simulink model "VSI_o_loop_Gid"  (Simulink 8.2)
settings: Solver=ode23t  StartTime=0.0  StopTime=0.5  MaxStep=25e-6  RelTol=1e-4  AbsTol=1e-5
values from neighbouring files (symbols this model uses):
  C = 1*31.5e-6    (= 3.15e-05)    [TVSI_vil_tf_cal_sim_comp_frd_model.m]    (also in VSI_ol_init.m = 3.13e-05; VSI_ol_tf_cal_sim_comp_frd_model.m = 3.13e-05; Zac_VSI.m = 3.18e-05; Zdc_VSI.m)
  Dd = 0.29997    [TVSI_vil_tf_cal_sim_comp_frd_model.m]    (also in VSI_ol_init.m = 0.299645524555; VSI_ol_tf_cal_sim_comp_frd_model.m = 0.367252524302; Zac_VSI.m = 0.3674)
  Dq = 0.08    [TVSI_vil_tf_cal_sim_comp_frd_model.m]    (also in VSI_ol_init.m = 0.0661607498065; VSI_ol_tf_cal_sim_comp_frd_model.m = 0.000664512470614; Zac_VSI.m = 0.0012)
  L = 1.0e-3    (= 0.001)    [TVSI_vil_tf_cal_sim_comp_frd_model.m]    (also in VSI_ol_init.m; VSI_ol_tf_cal_sim_comp_frd_model.m; Zac_VSI.m = 0.000506643235509; Zdc_VSI.m)
  R = 12    [TVSI_vil_tf_cal_sim_comp_frd_model.m]    (also in VSI_ol_init.m = 15; VSI_ol_tf_cal_sim_comp_frd_model.m = 12000; Zac_VSI.m; Zdc_VSI.m)
  RL = 0.13    [TVSI_vil_tf_cal_sim_comp_frd_model.m]    (also in VSI_ol_init.m = 0.15; VSI_ol_tf_cal_sim_comp_frd_model.m = 0.15; Zac_VSI.m = 0.06; Zdc_VSI.m)
  Vdc = 270    [TVSI_vil_tf_cal_sim_comp_frd_model.m]    (also in VSI_ol_init.m; VSI_ol_tf_cal_sim_comp_frd_model.m; Zac_VSI.m; Zdc_VSI.m)
  w = 500*2*pi    (= 3141.59265359)    [JF_CMOD.m]    (also in JF_SMOD.m; TVSI_vil_tf_cal_sim_comp_frd_model.m = 376.991118431; VSI_ol_init.m = 2513.27412287; VSI_ol_tf_cal_sim_comp_frd_model.m = 376.991118431)
libraries: powerlib x22
settings Model: Creator=marko  LastModifiedBy=wenbo  BufferReuse=off
settings OptimizationCC: BlockReduction=off  InlineParams=on  BufferReuse=off
settings DebuggingCC: AlgebraicLoopMsg=none  SolverPrmCheckMsg=none  UnconnectedInputMsg=none  UnconnectedOutputMsg=none  UnconnectedLineMsg=none

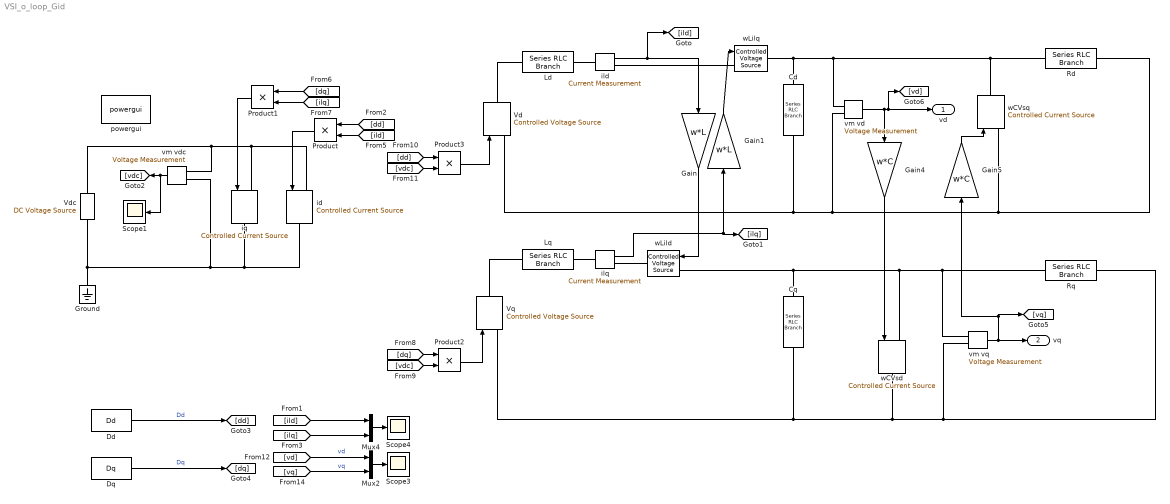
== system VSI_o_loop_Gid ==
  Cd : powerlib/Elements/Series RLC Branch  LConnTagsString=__new0  RConnTagsString=__new0  BranchType=C  Resistance=1  Inductance=1e-3  SetiL0=off  InitialCurrent=0  Capacitance=C  Setx0=off  InitialVoltage=0  Measurements=None
  Cq : powerlib/Elements/Series RLC Branch  LConnTagsString=__new0  RConnTagsString=__new0  BranchType=C  Resistance=1  Inductance=1e-3  SetiL0=off  InitialCurrent=0  Capacitance=C  Setx0=off  InitialVoltage=0  Measurements=None
  Dd : Constant  Value=Dd
  Dq : Constant  Value=Dq
  Gain : Gain  Gain=w*L
  Gain1 : Gain  Gain=w*L
  Gain4 : Gain  Gain=w*C
  Gain5 : Gain  Gain=w*C
  Ground : powerlib/Elements/Ground  LConnTagsString=a
  Ld : powerlib/Elements/Series RLC Branch  LConnTagsString=__new0  RConnTagsString=__new0  BranchType=RL  Resistance=RL  Inductance=L  SetiL0=off  InitialCurrent=0  Capacitance=1e-6  Setx0=off  InitialVoltage=0  Measurements=None
  Lq : powerlib/Elements/Series RLC Branch  LConnTagsString=__new0  RConnTagsString=__new0  BranchType=RL  Resistance=RL  Inductance=L  SetiL0=off  InitialCurrent=0  Capacitance=1e-6  Setx0=off  InitialVoltage=0  Measurements=None
  Mux2 : Mux  Inputs=2
  Mux4 : Mux  Inputs=2
  Product{,1..3} (4 alike) : Product  RndMeth=Zero
  Rd : powerlib/Elements/Series RLC Branch  LConnTagsString=__new0  RConnTagsString=__new0  BranchType=R  Resistance=R  Inductance=1e-3  SetiL0=off  InitialCurrent=0  Capacitance=1e-6  Setx0=off  InitialVoltage=0  Measurements=None
  Rq : powerlib/Elements/Series RLC Branch  LConnTagsString=__new0  RConnTagsString=__new0  BranchType=R  Resistance=R  Inductance=1e-3  SetiL0=off  InitialCurrent=0  Capacitance=1e-6  Setx0=off  InitialVoltage=0  Measurements=None
  Scope1 : Scope
      settings: YMin=270  YMax=270  SaveName=ildq_matlab
  Scope3 : Scope
      settings: YMin=-0.25  YMax=5.25  SaveName=ildq_matlab2
  Scope4 : Scope
      settings: YMin=-0.25  YMax=5.25  SaveName=ildq_matlab1
  Vd : powerlib/Electrical Sources/Controlled Voltage Source  Initialize=on  Source_Type=DC  Amplitude=0  Phase=0  Frequency=0  Measurements=None
  Vdc : powerlib/Electrical Sources/DC Voltage Source  Amplitude=Vdc  Measurements=None
  Vq : powerlib/Electrical Sources/Controlled Voltage Source  Initialize=on  Source_Type=DC  Amplitude=0  Phase=0  Frequency=0  Measurements=None
  id : powerlib/Electrical Sources/Controlled Current Source  Initialize=on  Source_Type=DC  Amplitude=0  Phase=0  Frequency=0  Measurements=None
  ild : powerlib/Measurements/Current Measurement  PhasorSimulation=off  OutputType=Complex  PSBequivalent=0
  ilq : powerlib/Measurements/Current Measurement  PhasorSimulation=off  OutputType=Complex  PSBequivalent=0
  iq : powerlib/Electrical Sources/Controlled Current Source  Initialize=on  Source_Type=DC  Amplitude=0  Phase=0  Frequency=0  Measurements=None
  powergui : powerlib/powergui  Priority=1  SimulationMode=Continuous  SolverType=Tustin  SampleTime=50e-6  frequency=60  SPID=off  DisableSnubberDevices=off  DisableRonSwitches=off  DisableVfSwitches=off  SwTol=0  Interpol=off  DisplayEquations=off  frequencyindice=0  Pbase=100e6  ErrMax=1e-4  Iterations=50  UnitsV=kV  UnitsW=MW  FunctionMessages=off  echomessages=off  HookPort=off  EnableUseOfTLC=off  x0status=blocks  RestoreLinks=warning  ResistiveCurrentMeasurement=off  Frange=[0:2:500]  Ylog=off  Xlog=on  ShowGrid=off  save=off  variable=ZData  ZoomFFT=on  StartTime=0.0  cycles=1  DisplayStyle=1  fundamental=60  FreqAxis=off  MaxFrequency=1000  frequencyindicesteady=1  RmsSteady=1  display=off  Ts=0  methode=off
  vm vd : powerlib/Measurements/Voltage Measurement  PhasorSimulation=off  OutputType=Complex  PSBequivalent=0
  vm vdc : powerlib/Measurements/Voltage Measurement  PhasorSimulation=off  OutputType=Complex  PSBequivalent=0
  vm vq : powerlib/Measurements/Voltage Measurement  PhasorSimulation=off  OutputType=Complex  PSBequivalent=0
  wCVsd : powerlib/Electrical Sources/Controlled Current Source  Initialize=on  Source_Type=DC  Amplitude=0  Phase=0  Frequency=0  Measurements=None
  wCVsq : powerlib/Electrical Sources/Controlled Current Source  Initialize=on  Source_Type=DC  Amplitude=0  Phase=0  Frequency=0  Measurements=None
  wLild : powerlib/Electrical Sources/Controlled Voltage Source  Initialize=on  Source_Type=DC  Amplitude=0  Phase=0  Frequency=0  Measurements=None
  wLilq : powerlib/Electrical Sources/Controlled Voltage Source  Initialize=on  Source_Type=DC  Amplitude=0  Phase=0  Frequency=0  Measurements=None
  vd : Outport
  vq : Outport  Port=2
  wires:
  Product1/1 -> iq/1
  [dq] -> Product2/1
  [vdc] -> Product2/2
  Product2/1 -> Vq/1
  [dd] -> Product3/1
  [vdc] -> Product3/2
  Product3/1 -> Vd/1
  vm vd/1 -> vd/1, [vd], Gain4/1
  vm vq/1 -> vq/1, Gain5/1, [vq]
  vm vdc/1 -> [vdc], Scope1/1
  ilq/1 -> [ilq], Gain1/1
  ild/1 -> Gain/1, [ild]
  Gain5/1 -> wCVsq/1
  [ild] -> Mux4/1
  [ilq] -> Mux4/2
  Mux4/1 -> Scope4/1
  [vd] -> Mux2/1  "vd"
  [vq] -> Mux2/2  "vq"
  Mux2/1 -> Scope3/1
  Dd/1 -> [dd]  "Dd"
  Dq/1 -> [dq]  "Dq"
  [dd] -> Product/1
  [ild] -> Product/2
  [dq] -> Product1/1
  [ilq] -> Product1/2
  Product/1 -> id/1
  Gain/1 -> wLild/1
  Gain1/1 -> wLilq/1
  Gain4/1 -> wCVsd/1
  connections:
  wCVsd/RConn1 -- Rq/RConn1 -- vm vq/LConn2 -- Cq/RConn1 -- Vq/LConn1
  vm vdc/LConn2 -- id/RConn1 -- iq/RConn1 -- Ground/LConn1 -- Vdc/LConn1
  Cq/LConn1 -- wCVsd/LConn1 -- Rq/LConn1 -- vm vq/LConn1 -- wLild/LConn1
  wLild/RConn1 -- ilq/RConn1
  ilq/LConn1 -- Lq/LConn1
  Lq/RConn1 -- Vq/RConn1
  Vdc/RConn1 -- vm vdc/LConn1 -- iq/LConn1 -- id/LConn1
  wLilq/RConn1 -- wCVsq/RConn1 -- Rd/LConn1 -- vm vd/LConn1 -- Cd/LConn1
  ild/LConn1 -- Ld/RConn1
  Ld/LConn1 -- Vd/RConn1
  wLilq/LConn1 -- ild/RConn1
  Cd/RConn1 -- wCVsq/LConn1 -- Rd/RConn1 -- vm vd/LConn2 -- Vd/LConn1
